simulink model "frequency_sim"  (Simulink 7.5)
settings: Solver=ode45  StartTime=0.0  StopTime=5  RelTol=1e-3
StopFcn:
  | save_system(vars.simfilename);
CloseFcn:
  | save_system(vars.simfilename); sim(vars.simfilename);vars.simtime = str2num(get_param(vars.simfilename,'StopTime'));set(guiel.hSimtime,'String',num2str(vars.simtime));if strcmp(vars.simfilename(end-2:end),'sim') vars.L= motorParams(1,1); vars.R= motorParams(1,2); vars.J= motorParams(1,3);vars.b= motorParams(1,4); vars.Kb= motorParams(1,5); vars.Km= motorParams(1,6);if (min(size(motorParams)) == 9) vars.P= motorParams(1,7); vars.I= motorParams(1,8); vars.D= motorParams(1,9);else;vars.P= NaN; vars.I= NaN; vars.D= NaN;end;clear motorParams; [vars.numericTF vars.symbolTF] = calcTF2(vars);end,
settings Model: Creator=Dan  LastModifiedBy=Dan
settings DataIOCC: MaxDataPoints=10000
settings OptimizationCC: BlockReduction=off  BooleanDataType=off  InitFltsAndDblsToZero=on
settings DebuggingCC: SaveWithParameterizedLinksMsg=none  SignalResolutionControl=TryResolveAllWithWarning  SolverPrmCheckMsg=none  MultiTaskDSMMsg=warning  MultiTaskCondExecSysMsg=none  StrictBusMsg=None
settings HardwareCC: TargetUnknown=on
settings RTWCC: IncludeERTFirstTime=on
settings GRTTargetCC: TargetFcnLib=ansi_tfl_tmw.mat

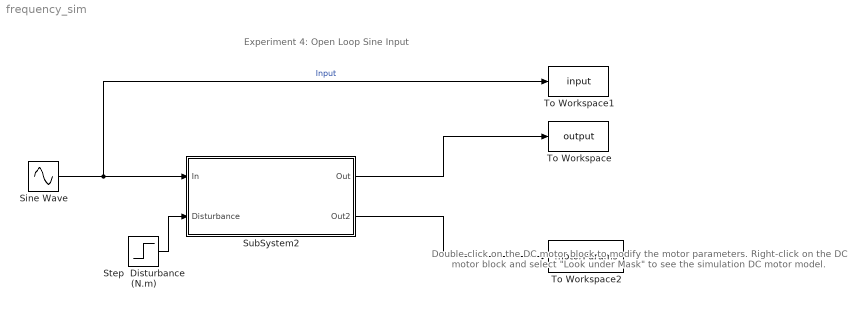
== system frequency_sim ==
  note: Experiment 4: Open Loop Sine Input
  note: Double-click on the
      | DC motor block to modify
      | the motor parameters.
      |
      | Right-click on the DC motor
      | block and select "Look under
      | Mask" to see the simulation
      | DC motor model.
  Sine Wave : Sin  Amplitude=20  Bias=0  Frequency=50  Phase=0  Samples=10  SampleTime=0  Offset=0
  Step  Disturbance (N.m) : Step  Time=0  After=0  SampleTime=0
  SubSystem2 : Subsystem  mask{L=0.00056, R=1.35, J=0.0019, b=0.000792, Kb=0.10, Km=0.10}
      mask prompts: L "Armature Inductance (L [H])"; R "Armature Resistance (R [ohm])"; J "Motor and Load Inertia (J [kg.m^2])"; b "Viscous damping friction (b[kg.m^2/s])"; Kb "Back emf constant (Kb [V/rad/s])"; Km "Motor constant (Km [N.m/A])"
      mask Display: disp('DC Motor (Speed Output)')
  To Workspace : ToWorkspace  VariableName=output  SampleTime=-1  SaveFormat=Structure With Time
  To Workspace1 : ToWorkspace  VariableName=input  SampleTime=-1  SaveFormat=Structure With Time
  To Workspace2 : ToWorkspace  VariableName=motorParams  SampleTime=-1  SaveFormat=Array
  wires:
  Sine Wave/1 -> To Workspace1/1, SubSystem2/1(In)  "Input"
  Step  Disturbance (N.m)/1 -> SubSystem2/2(Disturbance)
  SubSystem2/2(Out2) -> To Workspace2/1
  SubSystem2/1(Out) -> To Workspace/1

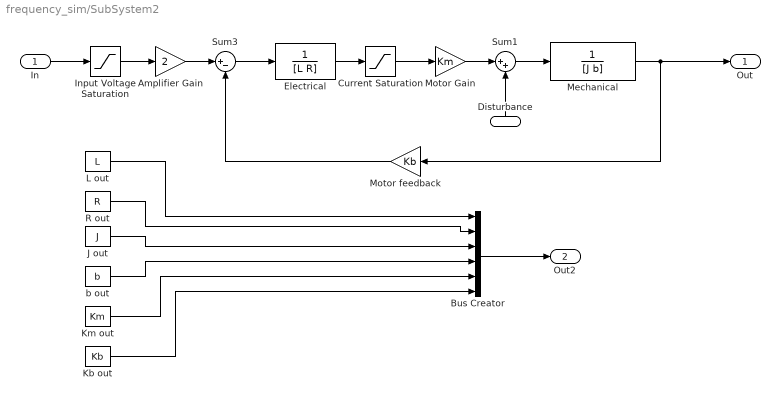
== system frequency_sim/SubSystem2 ==
  In : Inport  OutDataType=sfix(16)  OutScaling=2^0
  Disturbance : Inport  Port=2  OutDataType=sfix(16)  OutScaling=2^0
  Amplifier Gain : Gain  Gain=2  ParameterDataType=sfix(16)  ParameterScaling=2^0  OutDataType=sfix(16)  OutScaling=2^0  SaturateOnIntegerOverflow=on  OutDataTypeStr=Inherit: Same as input  ParamDataTypeStr=Inherit: Same as input
  Bus Creator : BusCreator  Inputs=6
  Current Saturation : Saturate  UpperLimit=+4  LowerLimit=-4
  Electrical : TransferFcn  Denominator=[L R]
  Input Voltage Saturation : Saturate  UpperLimit=+10  LowerLimit=-10
  J out : Constant  Value=J  OutDataType=sfix(16)  OutScaling=2^0
  Kb out : Constant  Value=Kb  OutDataType=sfix(16)  OutScaling=2^0
  Km out : Constant  Value=Km  OutDataType=sfix(16)  OutScaling=2^0
  L out : Constant  Value=L  OutDataType=sfix(16)  OutScaling=2^0
  Mechanical : TransferFcn  Denominator=[J b]
  Motor Gain : Gain  Gain=Km  ParameterDataType=sfix(16)  ParameterScaling=2^0  OutDataType=sfix(16)  OutScaling=2^0  SaturateOnIntegerOverflow=on  OutDataTypeStr=Inherit: Same as input  ParamDataTypeStr=Inherit: Same as input
  Motor feedback : Gain  Gain=Kb  ParameterDataType=sfix(16)  ParameterScaling=2^0  OutDataType=sfix(16)  OutScaling=2^0  SaturateOnIntegerOverflow=on  OutDataTypeStr=Inherit: Same as input  ParamDataTypeStr=Inherit: Same as input
  R out : Constant  Value=R  OutDataType=sfix(16)  OutScaling=2^0
  Sum1 : Sum  Inputs=|++  OutDataType=sfix(16)  OutScaling=2^0  SaturateOnIntegerOverflow=on  InputSameDT=on  OutDataTypeStr=Inherit: Same as first input
  Sum3 : Sum  Inputs=|+-  OutDataType=sfix(16)  OutScaling=2^0  SaturateOnIntegerOverflow=on  InputSameDT=on  OutDataTypeStr=Inherit: Same as first input
  b out : Constant  Value=b  OutDataType=sfix(16)  OutScaling=2^0
  Out : Outport  OutDataType=sfix(16)  OutScaling=2^0
  Out2 : Outport  Port=2  OutDataType=sfix(16)  OutScaling=2^0
  wires:
  Disturbance/1 -> Sum1/2
  Motor Gain/1 -> Sum1/1
  Sum1/1 -> Mechanical/1
  Motor feedback/1 -> Sum3/2
  Electrical/1 -> Current Saturation/1
  Mechanical/1 -> Out/1, Motor feedback/1
  Sum3/1 -> Electrical/1
  In/1 -> Input Voltage Saturation/1
  Amplifier Gain/1 -> Sum3/1
  Input Voltage Saturation/1 -> Amplifier Gain/1
  Current Saturation/1 -> Motor Gain/1
  L out/1 -> Bus Creator/1
  R out/1 -> Bus Creator/2
  J out/1 -> Bus Creator/3
  b out/1 -> Bus Creator/4
  Km out/1 -> Bus Creator/5
  Kb out/1 -> Bus Creator/6
  Bus Creator/1 -> Out2/1
